simulink model "Smart_Inverter_Toolbox"  (R2024a)
settings: Solver=ode4  StartTime=0.0  StopTime=10.0  FixedStep=50e-6  RelTol=1e-3
undefined symbols (not defined in the file): DiscIntNeverNeededParam
libraries: simulink x4, spsFirstOrderFilterLib x4, spsThreePhaseSeriesRLCBranchLib x4, spsControlledVoltageSourceLib x3, spsGroundLib x2, slpidlib x2, spsabctodq0Lib x2, spsThreePhaseVIMeasurementLib x2, eeGeneralControl x1, spsdq0toabcLib x1, spsThreePhaseSourceLib x1, sps_lib x1
settings Model: Creator=Gokul_SENTRY  LastModifiedBy=Gokul_SENTRY

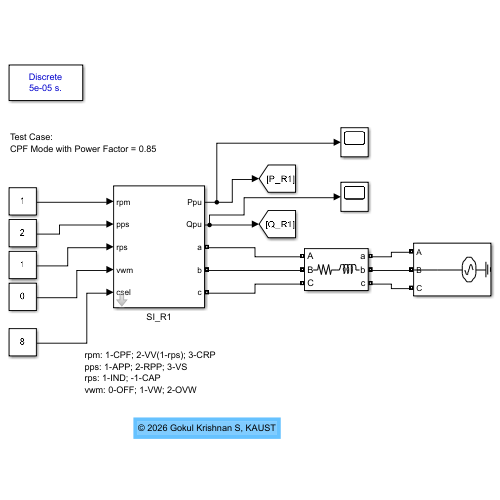
[thumbnail: Simulink's stored preview of the top-level diagram]
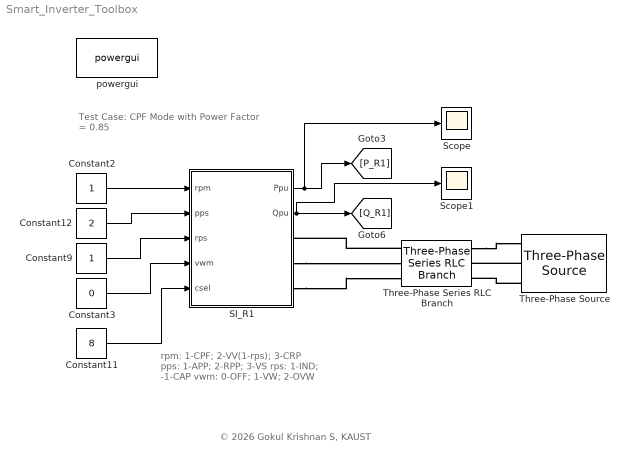
== system Smart_Inverter_Toolbox ==
  note: © 2026 Gokul Krishnan S, KAUST
  note: Test Case:
      | CPF Mode with Power Factor = 0.85
  note: rpm: 1-CPF; 2-VV(1-rps); 3-CRP
      | pps: 1-APP; 2-RPP; 3-VS
      | rps: 1-IND; -1-CAP
      | vwm: 0-OFF; 1-VW; 2-OVW
  Constant11 : Constant  Value=8
  Constant12 : Constant  Value=2
  Constant2 : Constant
  Constant3 : Constant  Value=0
  Constant9 : Constant
  SI_R1 : Subsystem  mask{Sb=10e3, Vb=400, Freq=50, rpm=CPF, pps=Active Power Priority, rps=Inductive, vwm=Off}
      mask prompts: Sb "Rated Power (VA)"; Vb "Ph-Ph RMS Voltage (V)"; Freq "Frequency (Hz)"; rpm "Reactive Power Mode"; pps "Power Priority"; rps "Reactive Power"; vwm "Volt-Watt Mode"
      mask init:
      | Idr_p = 10;      % Inductor Current Ripple in %
      | Ma    = 0.84;    % Modulation Index
      | Fsw   = 10e3;    % Inverter switching frequency (Hz)
      | Ka_p  = 20;      % Attenuation factor in %
      | 
      | Zb = (Vb^2)/Sb;
      | Cb = 1/(2*pi*Freq*Zb);
      | Vdc = (2*Vb*sqrt(2))/(Ma*sqrt(3));
      | Ib = Sb/(sqrt(3)*Vb);
      | Ib_max = Ib*sqrt(2);
      | Ir_max = Ib_max*(Idr_p/100);
      | Ka = Ka_p/100;
      | 
      | Cf = Cb*0.01;
      | 
      | L1 = Vdc/(6*Fsw*Ir_max);
      | L2 = ((sqrt(1/Ka^2))+1)/(Cf*((2*pi*Fsw)^2));
      | 
      | Fres = (1/(2*pi))*sqrt((L1+L2)/(L1*L2*Cf));
      | Rf   = 1/(3*Cf*Fres*2*pi);
      | 
      | CDC_bus = ((4*Sb)/(Vdc^2))*(1/(4*Freq));
      | 
      | PLL_Kp = -2/(Vb*sqrt(2)*(1/4)*(1/Freq));
      | PLL_Ki = PLL_Kp/(2*(1/4)*(1/Freq));
      | 
      | CC_Kp = (2*(L1+L2))/(1e-3);
      | CC_Ki = CC_Kp/(2*1e-3);
      mask TypeOptions rpm: CPF | VV | CRP
      mask TypeOptions pps: Active Power Priority | Reactive Power Priority | Vector Scaling
      mask DialogControl DescGroupVar Prompt: Smart Inverter Toolbox
      mask DialogControl DescTextVar Prompt: by Gokul, ANGLE Lab, KAUST
  Scope : Scope
  Scope1 : Scope
  Three-Phase Series RLC Branch : spsThreePhaseSeriesRLCBranchLib/Three-Phase Series RLC Branch  LConnTagsString=A|B|C  RConnTagsString=A|B|C  BranchType=RL  Resistance=1e-3  Inductance=1e-6  Capacitance=1e-6  Measurements=None
  Three-Phase Source : spsThreePhaseSourceLib/Three-Phase Source  InternalConnection=Yg  VoltagePhases=off  Voltage=400  PhaseAngle=0  Voltage_phases=[25e3 25e3 25e3]/sqrt(3)  PhaseAngles_phases=[0 -120 +120]  Frequency=50  NonIdealSource=off  SpecifyImpedance=off  Resistance=0.8929  Inductance=16.58e-3  ShortCircuitLevel=100e6  BaseVoltage=25e3  XRratio=7  BusType=swing  Pref=10e3  Qref=0  Prefabc=[10e3, 10e3, 10e3]  Qrefabc=[0, 0, 0]  Qmin=-inf  Qmax=inf
  powergui : sps_lib/powergui  Priority=1  SimulationMode=Discrete  SampleTime=50e-6  frequency=60  Iterations=50  frequencyindice=50  Pbase=100e6  ErrMax=1e-4  UnitsV=kV  UnitsW=MW  buscounter=0  FunctionMessages=off  echomessages=off  EnableUseOfTLC=off  CurrentSourceSwitches=off  DisableSnubberDevices=off  DisableRonSwitches=off  DisableVfSwitches=off  DisplayEquations=off  AutomaticDiscreteSolvers=off  SolverType=Tustin/Backward Euler (TBE)  Interpol=off  ExternalGateDelay=off  methode=off  Ts=100  x0status=blocks  SPID=on  SwTol=0  HookPort=off  NonlinearTolerance=1e-4  nMaxIteration=100  ContinueOnMaxIteration=off  RestoreLinks=warning  ResistiveCurrentMeasurement=off  Frange=[0:2:500]  Ylog=off  Xlog=on  ShowGrid=off  save=off  variable=ZData  structure=0  ZoomFFT=off  StartTime=0.0  cycles=1  DisplayStyle=1  fundamental=60  FreqAxis=off  MaxFrequency=1000  frequencyindicesteady=1  RmsSteady=1  display=off
  wires:
  Constant9/1 -> SI_R1/3(rps)
  Constant12/1 -> SI_R1/2(pps)
  SI_R1/1(Ppu) -> Scope/1, [P_R1]
  Constant3/1 -> SI_R1/4(vwm)
  Constant11/1 -> SI_R1/5(csel)
  Constant2/1 -> SI_R1/1(rpm)
  SI_R1/2(Qpu) -> Scope1/1, [Q_R1]
  connections:
  SI_R1/RConn2 -- Three-Phase Series RLC Branch/LConn2
  Three-Phase Series RLC Branch/LConn1 -- SI_R1/RConn1
  SI_R1/RConn3 -- Three-Phase Series RLC Branch/LConn3
  Three-Phase Source/RConn2 -- Three-Phase Series RLC Branch/RConn2
  Three-Phase Series RLC Branch/RConn1 -- Three-Phase Source/RConn1
  Three-Phase Source/RConn3 -- Three-Phase Series RLC Branch/RConn3

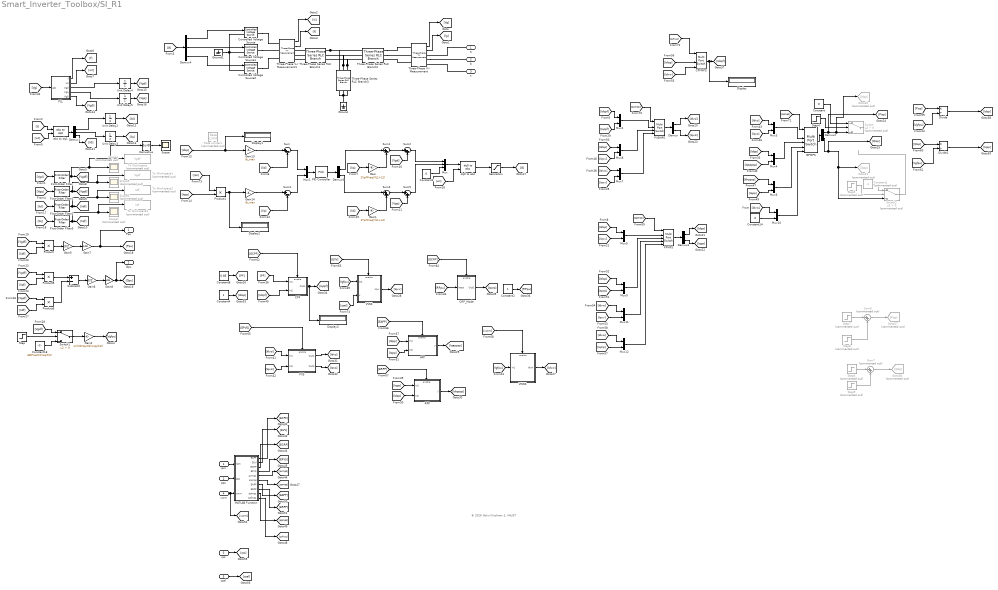
== system Smart_Inverter_Toolbox/SI_R1 ==
  note: © 2026 Gokul Krishnan S, KAUST
  rpm : Inport
  pps : Inport  Port=2
  rps : Inport  Port=3
  vwm : Inport  Port=4
  csel : Inport  Port=5
  APP : Subsystem
  CPF : Subsystem
  CPFMPS : MultiPortSwitch  DataPortOrder=Zero-based contiguous  zeroidx=on  SaturateOnIntegerOverflow=off  InputSameDT=off
  CRP_Mode : Subsystem
  Constant : Constant  Value=0
  Constant1 : Constant  Commented=on  Value=-1
  Constant14 : Constant  Value=0
  Constant18 : Constant  Value=400*sqrt(2)/sqrt(3)
  Constant2 : Constant
  Constant3 : Constant  Value=0
  Constant4 : Constant
  Constant8 : Constant  Value=0.85
  Controlled Voltage Source : spsControlledVoltageSourceLib/Controlled Voltage Source  Initialize=off  Source_Type=AC  Amplitude=0  Phase=0  Frequency=0  Measurements=None
  Controlled Voltage Source1 : spsControlledVoltageSourceLib/Controlled Voltage Source  Initialize=off  Source_Type=AC  Amplitude=0  Phase=0  Frequency=0  Measurements=None
  Controlled Voltage Source2 : spsControlledVoltageSourceLib/Controlled Voltage Source  Initialize=off  Source_Type=AC  Amplitude=0  Phase=0  Frequency=0  Measurements=None
  Demux{,2..3,9} (4 alike) : Demux  Outputs=2
  Demux1 : Demux  Outputs=3
  Demux4 : Demux  Outputs=3
  Derivative : Derivative
  Display{,1..3} (4 alike) : Display
  Divide : Product  Inputs=*/
  Divide1 : Product  Inputs=*/
  First-Order Filter : spsFirstOrderFilterLib/First-Order Filter  FilterType=Lowpass  Tc=10e-3  Ts=0  Initialize=on  Vac_Init=[((Vb*sqrt(2))/sqrt(3)), 0, Freq]  Vdc_Init=0  PlotResponse=off  FreqRange="[0,  200,  1]"
  First-Order Filter1 : spsFirstOrderFilterLib/First-Order Filter  FilterType=Lowpass  Tc=10e-3  Ts=0  Initialize=on  Vac_Init=[0, 0, Freq]  Vdc_Init=0  PlotResponse=off  FreqRange="[0,  200,  1]"
  First-Order Filter2 : spsFirstOrderFilterLib/First-Order Filter  FilterType=Lowpass  Tc=10e-3  Ts=0  Initialize=on  Vac_Init=[0, 0, Freq]  Vdc_Init=0  PlotResponse=off  FreqRange="[0,  200,  1]"
  First-Order Filter3 : spsFirstOrderFilterLib/First-Order Filter  FilterType=Lowpass  Tc=10e-3  Ts=0  Initialize=on  Vac_Init=[0, 0, Freq]  Vdc_Init=0  PlotResponse=off  FreqRange="[0,  200,  1]"
  Gain : Gain  Gain=2*pi*Freq*(L1+L2)
  Gain1 : Gain  Gain=2*pi*Freq*(L1+L2)
  Gain13 : Gain  Gain=Ib_max
  Gain14 : Gain  Gain=Ib_max
  Gain2 : Gain  Gain=1/((Vb*sqrt(2))/sqrt(3))
  Gain5 : Gain  Gain=3/2
  Gain6 : Gain  Gain=3/2
  Gain7 : Gain  Gain=1/Sb
  Gain8 : Gain  Gain=1/Sb
  Goto40 : Goto  Commented=on  GotoTag=Idsp
  Goto41 : Goto  Commented=on  GotoTag=Iqsp
  Goto57 : Goto  Commented=on  GotoTag=Pisp
  Goto58 : Goto  Commented=on  GotoTag=Qisp
  Ground : spsGroundLib/Ground  LConnTagsString=a
  Ground1 : spsGroundLib/Ground  LConnTagsString=a
  ISPMPS : MultiPortSwitch  DataPortOrder=Zero-based contiguous  Inputs=5  zeroidx=on  SaturateOnIntegerOverflow=off  InputSameDT=off
  MATLAB Function : MATLAB Function  TreatAsAtomicUnit=on
  Mux : Mux  Inputs=3
  Mux{1..12} (12 alike) : Mux  Inputs=2
  PID Controller : slpidlib/PID Controller  Controller=PI  Form=Parallel  TimeDomain=Continuous-time  UseExternalTs=off  SampleTime=-1  IntegratorMethod=Forward Euler  FilterMethod=Forward Euler  ControllerParametersSource=internal  P=CC_Kp  I=CC_Ki  UseKiTs=off  D=0  UseExternalDerivativeSource=off  N=100  UseFilter=on  TunerSelectOption=Transfer Function Based (PID Tuner App)  InitialConditionSource=internal  InitialConditionForIntegrator=0  InitialConditionForFilter=0  DifferentiatorICPrevScaledInput=0  ExternalReset=none  TrackingMode=off  Kt=1  LimitOutput=off  SatLimitsSource=internal  UpperSaturationLimit=inf  LowerSaturationLimit=-inf  LinearizeAsGain=on  AntiWindupMode=none  Kb=1  LimitIntegrator=off  UpperIntegratorSaturationLimit=inf  LowerIntegratorSaturationLimit=-inf  POutMin=[]  POutMax=[]  IOutMin=[]  IOutMax=[]  DOutMin=[]  DOutMax=[]  NOutMin=[]  NOutMax=[]  SumOutMin=[]  SumOutMax=[]  SaturationOutMin=[]  SaturationOutMax=[]  PParamMin=[]  PParamMax=[]  IParamMin=[]  IParamMax=[]  DParamMin=[]  DParamMax=[]  NParamMin=[]  NParamMax=[]  KbParamMin=[]  KbParamMax=[]  KtParamMin=[]  KtParamMax=[]  KbOutMin=[]  KbOutMax=[]  KtOutMin=[]  KtOutMax=[]  IntegratorOutMin=[]  IntegratorOutMax=[]  FilterOutMin=[]  FilterOutMax=[]  SumI1OutMin=[]  SumI1OutMax=[]  SumI2OutMin=[]  SumI2OutMax=[]  SumI3OutMin=[]  SumI3OutMax=[]  SumI4OutMin=[]  SumI4OutMax=[]  SumDOutMin=[]  SumDOutMax=[]  DifferentiatorOutMin=[]  DifferentiatorOutMax=[]  FilterDiffOutCoefMin=[]  FilterDiffOutCoefMax=[]  ReciprocalOutMin=[]  ReciprocalOutMax=[]  SumDenOutMin=[]  SumDenOutMax=[]  SumNumOutMin=[]  SumNumOutMax=[]  DivideOutMin=[]  DivideOutMax=[]  UdiffTsProdOutMin=[]  UdiffTsProdOutMax=[]  NTsProdOutMin=[]  NTsProdOutMax=[]  UintegralTsProdOutMin=[]  UintegralTsProdOutMax=[]  UngainTsProdOutMin=[]  UngainTsProdOutMax=[]  ClampingZeroOutDataTypeStr=Inherit: Inherit via back propagation  ClampingZeroOutMin=[]  ClampingZeroOutMax=[]  FilterDenConstantOutDataTypeStr=Inherit: Inherit via back propagation  FilterDenConstantOutMin=[]  FilterDenConstantOutMax=[]  PCopyOutDataTypeStr=Inherit: Inherit via back propagation  PCopyOutMin=[]  PCopyOutMax=[]  NCopyOutDataTypeStr=Inherit: Inherit via back propagation  NCopyOutMin=[]  NCopyOutMax=[]  IntegratorContinuousStateAttributes=''  IntegratorStateMustResolveToSignalObject=off  IntegratorRTWStateStorageClass=Auto  FilterContinuousStateAttributes=''  FilterStateMustResolveToSignalObject=off  FilterRTWStateStorageClass=Auto  ParallelPVariant=InternalParameters  IdealPVariant=Disabled  IVariant=InternalParameters  DVariant=Disabled  IntegratorVariant=Continuous  SatVariant=Disabled  AWVariant=Passthrough  PCopyVariant=Disabled  TRVariant=Disabled  FdbkBlocksVariant=Forward  IdealPFdbkVariant=Disabled  SatFdbkVariant=Disabled  DerivativeFilterVariant=Disabled  NVariant=Disabled  NCopyVariant=Disabled_SignalSpec  FilterICVariant=Disabled  IntegratorICVariant=InternalICs  ExternalResetVariant=Disabled  TRSumVariant=Passthrough  SumFdbkVariant=Disabled  SumVariant=Sum_PI  TsampFilterVariant=InternalTs  TsampNgainVariant=Passthrough  TsampIntegralVariant=Disabled_SignalSpec  ExternalSaturationOutDataTypeStr=Inherit: Same as second input  DerivativeSourceVariant=Disabled
  PLL : Subsystem
  PPMPS : MultiPortSwitch  DataPortOrder=Zero-based contiguous  Inputs=5  zeroidx=on  SaturateOnIntegerOverflow=off  InputSameDT=off
  PVS : Subsystem
  PVSMPS : MultiPortSwitch  DataPortOrder=Zero-based contiguous  Inputs=4  zeroidx=on  SaturateOnIntegerOverflow=off  InputSameDT=off
  Product{,1,5..6} (4 alike) : Product
  RPP : Subsystem
  Rate Limiter1 : RateLimiter  Commented=on  RisingSlewLimit=2  FallingSlewLimit=-2  SampleTimeMode=inherited
  Saturation : Saturate  UpperLimit=Vb*1.2*sqrt(2)/sqrt(3)  LowerLimit=-1*1.2*Vb*sqrt(2)/sqrt(3)
  Scope : Scope
  Scope{4..7} (4 alike) : Scope  Commented=on
  Step : Step  Time=0.1  SampleTime=0
  Step4 : Step  Time=7.05  SampleTime=0
  Step5 : Step  Commented=on  Time=7.05  SampleTime=0
  Step6 : Step  Commented=on  Time=3  Before=0.2  After=0.1  SampleTime=0
  Step7 : Step  Commented=on  Time=2  Before=0.9  After=0.8  SampleTime=0
  Step8 : Step  Commented=on  Time=2.5  After=+0.1  SampleTime=0
  Step9 : Step  Commented=on  Time=3.5  After=0.1  SampleTime=0
  Subtract2 : Sum  Inputs=+-
  Sum : Sum  Inputs=|+-
  Sum1 : Sum  Inputs=|+-
  Sum2 : Sum  Inputs=|++
  Sum3 : Sum  Inputs=|+-
  Sum4 : Sum  Inputs=|++
  Sum5 : Sum  Inputs=|++
  Sum6 : Sum  Commented=on  Inputs=|++
  Sum7 : Sum  Commented=on  Inputs=|++
  Switch : Switch  Commented=on  Criteria=u2 > Threshold  SaturateOnIntegerOverflow=off  InputSameDT=off
  Switch1 : Switch  Criteria=u2 > Threshold  SaturateOnIntegerOverflow=off  InputSameDT=off
  Switch2 : Switch  Commented=on  Criteria=u2 > Threshold  SaturateOnIntegerOverflow=off  InputSameDT=off
  Three-Phase Series RLC Branch1 : spsThreePhaseSeriesRLCBranchLib/Three-Phase Series RLC Branch  LConnTagsString=A|B|C  RConnTagsString=A|B|C  BranchType=L  Resistance=1  Inductance=L1  Capacitance=1e-6  Measurements=None
  Three-Phase Series RLC Branch2 : spsThreePhaseSeriesRLCBranchLib/Three-Phase Series RLC Branch  LConnTagsString=A|B|C  RConnTagsString=A|B|C  BranchType=L  Resistance=1  Inductance=L2  Capacitance=1e-6  Measurements=None
  Three-Phase Series RLC Branch3 : spsThreePhaseSeriesRLCBranchLib/Three-Phase Series RLC Branch  LConnTagsString=A|B|C  RConnTagsString=A|B|C  BranchType=RC  Resistance=Rf  Inductance=1e-3  Capacitance=Cf  Measurements=None
  Three-Phase V-I Measurement : spsThreePhaseVIMeasurementLib/Three-Phase V-I Measurement  VoltageMeasurement=phase-to-ground  SetLabelV=off  LabelV=Vabc  Vpu=off  VpuLL=off  CurrentMeasurement=yes  SetLabelI=off  LabelI=Iabc  Ipu=off  Pbase=100e6  Vbase=500e3  OutputType=Complex  PhasorSimulation=off  PSBequivalent=0
  Three-Phase V-I Measurement1 : spsThreePhaseVIMeasurementLib/Three-Phase V-I Measurement  VoltageMeasurement=phase-to-ground  SetLabelV=off  LabelV=Vabc  Vpu=off  VpuLL=off  CurrentMeasurement=yes  SetLabelI=off  LabelI=Iabc  Ipu=off  Pbase=100e6  Vbase=500e3  OutputType=Complex  PhasorSimulation=off  PSBequivalent=0
  To Workspace : ToWorkspace  Commented=on  VariableName=Vgdf  SaveFormat=Timeseries  SampleTime=-1
  To Workspace1 : ToWorkspace  Commented=on  VariableName=Vgqf  SaveFormat=Timeseries  SampleTime=-1
  To Workspace2 : ToWorkspace  Commented=on  VariableName=Iidf  SaveFormat=Timeseries  SampleTime=-1
  To Workspace3 : ToWorkspace  Commented=on  VariableName=Iiqf  SaveFormat=Timeseries  SampleTime=-1
  Unit Delay{2..5} (4 alike) : UnitDelay  SampleTime=-1  HasFrameUpgradeWarning=on
  VVSS : Subsystem
  VWSS : Subsystem
  abc to dq1 : spsabctodq0Lib/abc to dq0  Alignment=90 degrees behind phase A axis
  dq0 to abc : spsdq0toabcLib/dq0 to abc  Alignment=90 degrees behind phase A axis
  a : PMIOPort  Side=Right
  b : PMIOPort  Port=2  Side=Right
  c : PMIOPort  Port=3  Side=Right
  Ppu : Outport
  Qpu : Outport  Port=2
  wires:
  PLL/2(wt) -> [wt]
  [Iqsp] -> Product1/2
  Product1/1 -> Display2/1, Gain14/1
  MATLAB Function/10(cpfmps) -> [cpfmps]
  MATLAB Function/9(ppmps) -> [ppmps]
  MATLAB Function/8(ERPP) -> [ERPP]
  MATLAB Function/7(EAPP) -> [EAPP]
  MATLAB Function/6(spmps) -> [spmps]
  MATLAB Function/5(pvmps) -> [pvmps]
  MATLAB Function/4(EPVS) -> [EPVS]
  MATLAB Function/3(ECRP) -> [ECRP]
  MATLAB Function/2(EVV) -> [EVV]
  MATLAB Function/1(ECPF) -> [ECPF]
  vwm/1 -> MATLAB Function/3(vwm), [vwm]
  pps/1 -> MATLAB Function/2(pps)
  rpm/1 -> MATLAB Function/1(rpm)
  [Idsp] -> Display1/1, Gain13/1
  [Vgfpu] -> Divide/2
  Constant18/1 -> Switch1/3
  Step/1 -> Switch1/2
  [Vgdf] -> Switch1/1
  Switch1/1 -> Gain2/1
  [Vgfpu] -> Divide1/2
  [Qisp] -> Divide1/1
  [Pisp] -> Divide/1
  Saturation/1 -> [G]
  dq0 to abc/1 -> Saturation/1
  [Iqcrp] -> Mux12/2
  [Idvw] -> Mux12/1
  Mux12/1 -> PPMPS/6
  Unit Delay5/1 -> [Vgq]
  Unit Delay4/1 -> [Vgd]
  Unit Delay3/1 -> [Iiq]
  Unit Delay2/1 -> [Iid]
  [EPVS] -> PVS/Enable
  [ERPP] -> RPP/Enable
  [EAPP] -> APP/Enable
  [Idvw] -> CPFMPS/4
  [Idisp] -> CPFMPS/3
  [cpfmps] -> CPFMPS/1
  CPFMPS/1 -> Display/1, [Idcpf]
  Demux/1 -> [Idvsi]
  Mux7/1 -> PVSMPS/5
  [Iqvv] -> Mux7/2
  [Idvw] -> Mux7/1
  Mux11/1 -> PPMPS/5
  [Idvw] -> Mux11/1
  [Iqvv] -> Mux11/2
  Constant14/1 -> Mux10/2
  [Idvw] -> Mux10/1
  Mux10/1 -> ISPMPS/6
  Constant2/1 -> [RPpu]
  [Iqcrp] -> Mux9/2
  [Idisp] -> Mux9/1
  Mux9/1 -> PPMPS/4
  [vwm] -> VWSS/Enable
  [ECRP] -> CRP_Mode/Enable
  [EVV] -> VVSS/Enable
  [ECPF] -> CPF/Enable
  Mux5/1 -> PPMPS/3
  Mux6/1 -> ISPMPS/5
  Mux4/1 -> ISPMPS/4
  Mux3/1 -> ISPMPS/3
  Mux2/1 -> PVSMPS/3
  Mux8/1 -> PVSMPS/4
  [Idisp] -> Mux8/1
  [Iqvv] -> Mux8/2
  [Idrppsp] -> Mux6/1
  [Iqpp] -> Mux6/2
  [Iqvv] -> Mux5/2
  [Idisp] -> Mux5/1
  Demux3/2 -> [Iqpp]
  Demux3/1 -> [Idpp]
  PPMPS/1 -> Demux3/1
  [ppmps] -> PPMPS/1
  [Iqappsp] -> Mux4/2
  [Idpp] -> Mux4/1
  Constant4/1 -> [Idisp]
  Constant8/1 -> [PF]
  [spmps] -> ISPMPS/1
  ISPMPS/1 -> Demux2/1
  [Idvs] -> Mux3/1
  [Iqvs] -> Mux3/2
  [Iqcpf] -> Mux2/2
  [Idcpf] -> Mux2/1
  Demux/2 -> [Iqvsi]
  PVSMPS/1 -> Demux/1
  [pvmps] -> PVSMPS/1
  Gain5/1 -> Gain7/1
  [Iqpp] -> APP/2(In2)
  [Iqvsi] -> PVS/2(In2)
  [RPpu] -> CRP_Mode/1(Input)
  Gain8/1 -> [Qpu], Qpu/1
  First-Order Filter1/1 -> To Workspace1/1, Scope5/1, [Vgqf]
  VWSS/1(Idvw) -> [Idvw]
  Gain7/1 -> [Ppu], Ppu/1
  [wt] -> dq0 to abc/2
  [Vgdf] -> Product5/1
  PLL/4(Vgq) -> Unit Delay5/1
  PLL/5(Vg0) -> [Vg0]
  Three-Phase V-I Measurement/2 -> [Ig]
  Demux4/2 -> Controlled Voltage Source1/1
  [Vgq] -> First-Order Filter1/1
  [Idcpf] -> CPF/2(In2)
  CPF/1(Out1) -> Display3/1, [Iqcpf]
  First-Order Filter3/1 -> To Workspace3/1, Scope7/1, [Iiqf]
  [Vgfpu] -> VVSS/1(In1)
  [Idpp] -> APP/1(In1)
  [Iqpp] -> RPP/1(In1)
  APP/1(y) -> [Iqappsp]
  [Idpp] -> RPP/2(In2)
  [Iidf] -> Product6/2
  Gain6/1 -> Gain8/1
  First-Order Filter/1 -> Derivative/1, To Workspace/1, Scope4/1, [Vgdf]
  First-Order Filter2/1 -> To Workspace2/1, Scope6/1, [Iidf]
  [Iiqf] -> Product5/2
  PID Controller/1 -> Demux9/1
  Subtract2/1 -> Gain6/1
  CRP_Mode/1(Out1) -> [Iqcrp]
  [Iiq] -> Gain/1
  Product5/1 -> Subtract2/1
  [Vgfpu] -> VWSS/1(In1)
  Gain2/1 -> [Vgfpu]
  [Iiq] -> First-Order Filter3/1
  Sum/1 -> Mux1/1
  Three-Phase V-I Measurement/1 -> [Vg]
  Demux4/1 -> Controlled Voltage Source/1
  [Vgd] -> First-Order Filter/1
  [Vg] -> PLL/1(abc)
  Sum5/1 -> Mux/2
  [Vgq] -> Sum5/2
  PVS/2(Out2) -> [Iqvs]
  [Iid] -> Gain1/1
  Gain13/1 -> Sum/1
  Three-Phase V-I Measurement1/2 -> [Ii]
  RPP/1(y) -> [Idrppsp]
  [Iiq] -> Sum3/2
  Mux1/1 -> PID Controller/1
  [Ii] -> abc to dq1/1
  Demux1/2 -> Unit Delay3/1
  [Vgqf] -> Product6/1
  [Vgdf] -> Product/1
  Constant3/1 -> Mux/3
  abc to dq1/1 -> Demux1/1
  [G] -> Demux4/1
  [Iidf] -> Product/2
  Demux1/3 -> [Ii0]
  Mux/1 -> dq0 to abc/1
  Product6/1 -> Subtract2/2
  PVS/1(Out1) -> [Idvs]
  Sum1/1 -> Sum2/1
  [wt] -> abc to dq1/2
  [Idvsi] -> PVS/1(In1)
  Demux9/1 -> Sum1/1
  Sum2/1 -> Mux/1
  VVSS/1(Iqvv) -> [Iqvv]
  PLL/1(f) -> [f]
  Gain/1 -> Sum1/2
  Demux1/1 -> Unit Delay2/1
  Product/1 -> Gain5/1
  Demux9/2 -> Sum4/1
  [PF] -> CPF/1(In1)
  [Iid] -> Sum/2
  Sum4/1 -> Sum5/1
  [Iid] -> First-Order Filter2/1
  Gain1/1 -> Sum4/2
  PLL/3(Vgd) -> Unit Delay4/1
  [Vgd] -> Sum2/2
  Three-Phase V-I Measurement1/1 -> [Vi]
  Sum3/1 -> Mux1/2
  Demux4/3 -> Controlled Voltage Source2/1
  Divide/1 -> [Idsp]
  Divide1/1 -> [Iqsp]
  Derivative/1 -> Scope/1
  Gain14/1 -> Sum3/1
  Demux2/2 -> [Qisp], Switch2/3, Goto41/1
  Demux2/1 -> [Pisp], Switch/3, Goto40/1
  Constant/1 -> Switch/1
  Step4/1 -> Switch/2
  Step5/1 -> Switch2/2
  Switch2/1 -> ?
  Constant1/1 -> Switch2/1
  [rps] -> Product1/1
  rps/1 -> [rps]
  csel/1 -> [csel]
  [csel] -> VVSS/2(x)
  Sum7/1 -> Goto58/1
  Step8/1 -> Sum6/2
  Step9/1 -> Sum7/2
  Sum6/1 -> Goto57/1
  Step7/1 -> Sum6/1
  Step6/1 -> Sum7/1
  connections:
  Three-Phase V-I Measurement/RConn2 -- b/RConn1
  c/RConn1 -- Three-Phase V-I Measurement/RConn3
  Controlled Voltage Source1/LConn1 -- Controlled Voltage Source2/LConn1 -- Controlled Voltage Source/LConn1 -- Ground1/LConn1
  Three-Phase Series RLC Branch1/LConn2 -- Three-Phase V-I Measurement1/RConn2
  Three-Phase Series RLC Branch1/RConn1 -- Three-Phase Series RLC Branch3/LConn1 -- Three-Phase Series RLC Branch2/LConn1
  Three-Phase Series RLC Branch1/LConn1 -- Three-Phase V-I Measurement1/RConn1
  Three-Phase Series RLC Branch1/LConn3 -- Three-Phase V-I Measurement1/RConn3
  Three-Phase V-I Measurement/LConn3 -- Three-Phase Series RLC Branch2/RConn3
  Three-Phase Series RLC Branch2/RConn1 -- Three-Phase V-I Measurement/LConn1
  Controlled Voltage Source1/RConn1 -- Three-Phase V-I Measurement1/LConn2
  Three-Phase Series RLC Branch2/RConn2 -- Three-Phase V-I Measurement/LConn2
  Controlled Voltage Source2/RConn1 -- Three-Phase V-I Measurement1/LConn3
  a/RConn1 -- Three-Phase V-I Measurement/RConn1
  Three-Phase Series RLC Branch3/LConn2 -- Three-Phase Series RLC Branch1/RConn2 -- Three-Phase Series RLC Branch2/LConn2
  Controlled Voltage Source/RConn1 -- Three-Phase V-I Measurement1/LConn1
  Three-Phase Series RLC Branch3/LConn3 -- Three-Phase Series RLC Branch1/RConn3 -- Three-Phase Series RLC Branch2/LConn3
  Three-Phase Series RLC Branch3/RConn2 -- Ground/LConn1 -- Three-Phase Series RLC Branch3/RConn3 -- Three-Phase Series RLC Branch3/RConn1

== system Smart_Inverter_Toolbox/SI_R1/APP ==
  In1 : Inport
  In2 : Inport  Port=2
  Enable : EnablePort
  APP : simulink/Discontinuities/Saturation Dynamic  OutMin=[]  OutMax=[]  OutDataTypeStr=Inherit: Same as second input  OutDataType=fixdt(1, 16)  OutScaling=2^-10  DoSatur=off
  Constant25 : Constant
  Constant26 : Constant  Value=0
  Gain10 : Gain  Gain=-1
  Max2 : MinMax  Function=max  Inputs=2
  Square : Math  Operator=square
  Square Root : Sqrt
  Square1 : Math  Operator=square
  Subtract : Sum  Inputs=+-
  y : Outport
  wires:
  In1/1 -> Square1/1
  Subtract/1 -> Max2/1
  Square Root/1 -> Gain10/1, APP/1
  Constant26/1 -> Max2/2
  Max2/1 -> Square Root/1
  Square1/1 -> Subtract/2
  Gain10/1 -> APP/3
  In2/1 -> APP/2
  Square/1 -> Subtract/1
  APP/1 -> y/1
  Constant25/1 -> Square/1

== system Smart_Inverter_Toolbox/SI_R1/CPF ==
  In1 : Inport
  In2 : Inport  Port=2
  Enable : EnablePort
  Acos : Trigonometry  Operator=acos
  Product3 : Product
  Tan : Trigonometry  Operator=tan
  Out1 : Outport
  wires:
  Product3/1 -> Out1/1
  In1/1 -> Acos/1
  Tan/1 -> Product3/1
  In2/1 -> Product3/2
  Acos/1 -> Tan/1

== system Smart_Inverter_Toolbox/SI_R1/CRP_Mode ==
  Input : Inport
  Enable : EnablePort
  Constant2 : Constant
  Max1 : MinMax  Inputs=2
  Out1 : Outport
  wires:
  Max1/1 -> Out1/1
  Input/1 -> Max1/1
  Constant2/1 -> Max1/2

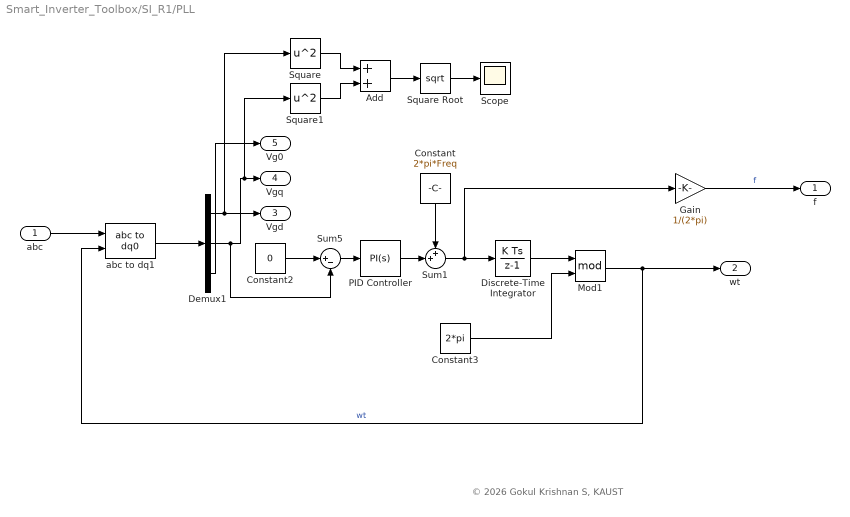
== system Smart_Inverter_Toolbox/SI_R1/PLL ==
  note: © 2026 Gokul Krishnan S, KAUST
  abc : Inport
  Add : Sum
  Constant : Constant  Value=2*pi*Freq
  Constant2 : Constant  Value=0
  Constant3 : Constant  Value=2*pi
  Demux1 : Demux  Outputs=3
  Discrete-Time Integrator : DiscreteIntegrator  SampleTime=-1  ICPrevOutput=DiscIntNeverNeededParam  ICPrevScaledInput=DiscIntNeverNeededParam
  Gain : Gain  Gain=1/(2*pi)
  Mod1 : Math  Operator=mod
  PID Controller : slpidlib/PID Controller  Controller=PI  Form=Parallel  TimeDomain=Continuous-time  UseExternalTs=off  SampleTime=-1  IntegratorMethod=Forward Euler  FilterMethod=Forward Euler  ControllerParametersSource=internal  P=PLL_Kp  I=PLL_Ki  UseKiTs=off  D=0  UseExternalDerivativeSource=off  N=100  UseFilter=on  TunerSelectOption=Transfer Function Based (PID Tuner App)  InitialConditionSource=internal  InitialConditionForIntegrator=0  InitialConditionForFilter=0  DifferentiatorICPrevScaledInput=0  ExternalReset=none  TrackingMode=off  Kt=1  LimitOutput=off  SatLimitsSource=internal  UpperSaturationLimit=inf  LowerSaturationLimit=-inf  LinearizeAsGain=on  AntiWindupMode=none  Kb=1  LimitIntegrator=off  UpperIntegratorSaturationLimit=inf  LowerIntegratorSaturationLimit=-inf  POutMin=[]  POutMax=[]  IOutMin=[]  IOutMax=[]  DOutMin=[]  DOutMax=[]  NOutMin=[]  NOutMax=[]  SumOutMin=[]  SumOutMax=[]  SaturationOutMin=[]  SaturationOutMax=[]  PParamMin=[]  PParamMax=[]  IParamMin=[]  IParamMax=[]  DParamMin=[]  DParamMax=[]  NParamMin=[]  NParamMax=[]  KbParamMin=[]  KbParamMax=[]  KtParamMin=[]  KtParamMax=[]  KbOutMin=[]  KbOutMax=[]  KtOutMin=[]  KtOutMax=[]  IntegratorOutMin=[]  IntegratorOutMax=[]  FilterOutMin=[]  FilterOutMax=[]  SumI1OutMin=[]  SumI1OutMax=[]  SumI2OutMin=[]  SumI2OutMax=[]  SumI3OutMin=[]  SumI3OutMax=[]  SumI4OutMin=[]  SumI4OutMax=[]  SumDOutMin=[]  SumDOutMax=[]  DifferentiatorOutMin=[]  DifferentiatorOutMax=[]  FilterDiffOutCoefMin=[]  FilterDiffOutCoefMax=[]  ReciprocalOutMin=[]  ReciprocalOutMax=[]  SumDenOutMin=[]  SumDenOutMax=[]  SumNumOutMin=[]  SumNumOutMax=[]  DivideOutMin=[]  DivideOutMax=[]  UdiffTsProdOutMin=[]  UdiffTsProdOutMax=[]  NTsProdOutMin=[]  NTsProdOutMax=[]  UintegralTsProdOutMin=[]  UintegralTsProdOutMax=[]  UngainTsProdOutMin=[]  UngainTsProdOutMax=[]  ClampingZeroOutDataTypeStr=Inherit: Inherit via back propagation  ClampingZeroOutMin=[]  ClampingZeroOutMax=[]  FilterDenConstantOutDataTypeStr=Inherit: Inherit via back propagation  FilterDenConstantOutMin=[]  FilterDenConstantOutMax=[]  PCopyOutDataTypeStr=Inherit: Inherit via back propagation  PCopyOutMin=[]  PCopyOutMax=[]  NCopyOutDataTypeStr=Inherit: Inherit via back propagation  NCopyOutMin=[]  NCopyOutMax=[]  IntegratorContinuousStateAttributes=''  IntegratorStateMustResolveToSignalObject=off  IntegratorRTWStateStorageClass=Auto  FilterContinuousStateAttributes=''  FilterStateMustResolveToSignalObject=off  FilterRTWStateStorageClass=Auto  ParallelPVariant=InternalParameters  IdealPVariant=Disabled  IVariant=InternalParameters  DVariant=Disabled  IntegratorVariant=Continuous  SatVariant=Disabled  AWVariant=Passthrough  PCopyVariant=Disabled  TRVariant=Disabled  FdbkBlocksVariant=Forward  IdealPFdbkVariant=Disabled  SatFdbkVariant=Disabled  DerivativeFilterVariant=Disabled  NVariant=Disabled  NCopyVariant=Disabled_SignalSpec  FilterICVariant=Disabled  IntegratorICVariant=InternalICs  ExternalResetVariant=Disabled  TRSumVariant=Passthrough  SumFdbkVariant=Disabled  SumVariant=Sum_PI  TsampFilterVariant=InternalTs  TsampNgainVariant=Passthrough  TsampIntegralVariant=Disabled_SignalSpec  ExternalSaturationOutDataTypeStr=Inherit: Same as second input  DerivativeSourceVariant=Disabled
  Scope : Scope
  Square : Math  Operator=square
  Square Root : Sqrt
  Square1 : Math  Operator=square
  Sum1 : Sum  Inputs=++|
  Sum5 : Sum  Inputs=|+-
  abc to dq1 : spsabctodq0Lib/abc to dq0  Alignment=90 degrees behind phase A axis
  f : Outport
  wt : Outport  Port=2
  Vgd : Outport  Port=3
  Vgq : Outport  Port=4
  Vg0 : Outport  Port=5
  wires:
  Square Root/1 -> Scope/1
  Add/1 -> Square Root/1
  Square1/1 -> Add/2
  Square/1 -> Add/1
  Constant2/1 -> Sum5/1
  Demux1/1 -> Vgd/1, Square/1
  Constant/1 -> Sum1/1
  Sum1/1 -> Discrete-Time Integrator/1, Gain/1
  PID Controller/1 -> Sum1/2
  Discrete-Time Integrator/1 -> Mod1/1
  Mod1/1 -> wt/1, abc to dq1/2  "wt"
  Demux1/2 -> Vgq/1, Square1/1, Sum5/2
  abc to dq1/1 -> Demux1/1
  Sum5/1 -> PID Controller/1
  Constant3/1 -> Mod1/2
  Demux1/3 -> Vg0/1
  abc/1 -> abc to dq1/1
  Gain/1 -> f/1  "f"

== system Smart_Inverter_Toolbox/SI_R1/PVS ==
  In1 : Inport
  In2 : Inport  Port=2
  Enable : EnablePort
  Add : Sum
  Constant29 : Constant
  Divide2 : Product  Inputs=*/
  Min : MinMax  Inputs=2
  Product1 : Product
  Product2 : Product
  Square Root2 : Sqrt
  Square4 : Math  Operator=square
  Square5 : Math  Operator=square
  Out1 : Outport
  Out2 : Outport  Port=2
  wires:
  Product2/1 -> Out2/1
  Product1/1 -> Out1/1
  Min/1 -> Product1/2, Product2/1
  Square5/1 -> Add/2
  In2/1 -> Square5/1, Product2/2
  Square4/1 -> Add/1
  Add/1 -> Square Root2/1
  Constant29/1 -> Divide2/1, Min/1
  Divide2/1 -> Min/2
  Square Root2/1 -> Divide2/2
  In1/1 -> Square4/1, Product1/1

== system Smart_Inverter_Toolbox/SI_R1/RPP ==
  In1 : Inport
  In2 : Inport  Port=2
  Enable : EnablePort
  Constant27 : Constant
  Constant28 : Constant  Value=0
  Gain11 : Gain  Gain=-1
  Max3 : MinMax  Function=max  Inputs=2
  RPP : simulink/Discontinuities/Saturation Dynamic  OutMin=[]  OutMax=[]  OutDataTypeStr=Inherit: Same as second input  OutDataType=fixdt(1, 16)  OutScaling=2^-10  DoSatur=off
  Square Root1 : Sqrt
  Square2 : Math  Operator=square
  Square3 : Math  Operator=square
  Subtract1 : Sum  Inputs=+-
  y : Outport
  wires:
  RPP/1 -> y/1
  In1/1 -> Square3/1
  Constant27/1 -> Square2/1
  Square2/1 -> Subtract1/1
  Square Root1/1 -> RPP/1, Gain11/1
  In2/1 -> RPP/2
  Max3/1 -> Square Root1/1
  Square3/1 -> Subtract1/2
  Subtract1/1 -> Max3/1
  Constant28/1 -> Max3/2
  Gain11/1 -> RPP/3

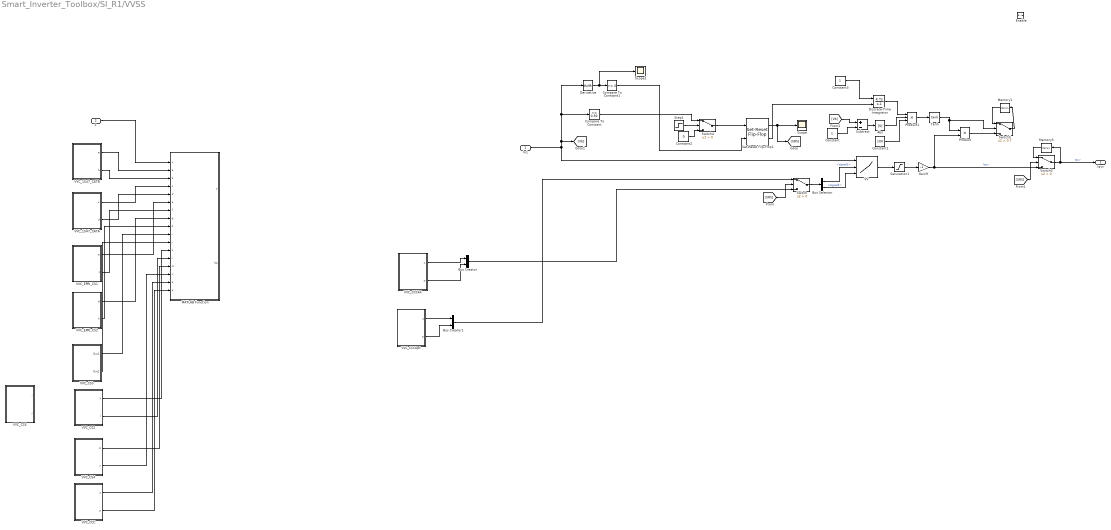
== system Smart_Inverter_Toolbox/SI_R1/VVSS ==
  In1 : Inport
  x : Inport  Port=2
  Enable : EnablePort
  Abs : Abs  SaturateOnIntegerOverflow=off
  Bus Creator : BusCreator  Inputs=2
  Bus Creator1 : BusCreator  Inputs=2
  Bus Selector : BusSelector  OutputSignals=signal1,signal2
  Compare To Constant : simulink/Logic and Bit Operations/Compare To Constant  relop=<=  const=0.92  OutDataTypeStr=boolean
  Compare To Constant1 : simulink/Logic and Bit Operations/Compare To Constant  relop=>=  const=4  OutDataTypeStr=boolean
  Constant : Constant
  Constant1 : Constant  Value=100
  Constant2 : Constant  Value=0
  Constant3 : Constant
  Derivative : Derivative
  Discrete-Time Integrator : DiscreteIntegrator  ExternalReset=level  SampleTime=-1  ICPrevOutput=DiscIntNeverNeededParam  ICPrevScaledInput=DiscIntNeverNeededParam
  Gain9 : Gain  Gain=-1
  MATLAB Function : MATLAB Function  TreatAsAtomicUnit=on
  Memory1 : Memory
  Memory3 : Memory
  Product : Product
  Product1 : Product  Inputs=3
  Saturation1 : Saturate  UpperLimit=1  LowerLimit=-1
  Scope : Scope
  Scope1 : Scope
  Set-Reset Flip-Flop1 : eeGeneralControl/Set-Reset Flip-Flop  LabelModeActiveChoice=Discrete  UndefState=Set  Q0=0  Ts=-1
      settings: LibrarySourceBlock=ee_sl_lib/General Control/Set-Reset Flip-Flop
  Step1 : Step  Time=2  SampleTime=0
  Subtract : Sum  Inputs=+-
  Switch : Switch  Criteria=u2 > Threshold  SaturateOnIntegerOverflow=off  InputSameDT=off
  Switch3 : Switch  Criteria=u2 > Threshold  SaturateOnIntegerOverflow=off  InputSameDT=off
  Switch4 : Switch  Criteria=u2 > Threshold  SaturateOnIntegerOverflow=off  InputSameDT=off
  Switch5 : Switch  Criteria=u2 > Threshold  Threshold=0.7  SaturateOnIntegerOverflow=off  InputSameDT=off
  Tanh : Trigonometry  Operator=tanh
  VV : Lookup_n-D  NumberOfTableDimensions=1  BreakpointsForDimension1Source=Input port  BreakpointsForDimension1=[-5:5]  TableSource=Input port  Table=tanh([-5:5])  ExtrapMethod=Clip  InternalRulePriority=Speed  RndMeth=Simplest
      settings: InputPortMap=u0,p221,p5
  VVC_1547_CATA : Subsystem
  VVC_1547_CATB : Subsystem
  VVC_CCC : Subsystem
  VVC_CCC44 : Subsystem
  VVC_CCCOpt : Subsystem
  VVC_CS2 : Subsystem
  VVC_CS3 : Subsystem
  VVC_CS4 : Subsystem
  VVC_CS5 : Subsystem
  VVC_EPRI_CS1 : Subsystem
  VVC_EPRI_CS2 : Subsystem
  Iqvv : Outport
  wires:
  x/1 -> MATLAB Function/1(x)
  VVC_1547_CATB/1(a) -> MATLAB Function/2(a)
  VVC_1547_CATB/2(b) -> MATLAB Function/3(b)
  VVC_1547_CATA/1(c) -> MATLAB Function/4(c)
  VVC_1547_CATA/2(d) -> MATLAB Function/5(d)
  VVC_EPRI_CS1/1(e) -> MATLAB Function/6(e)
  VVC_EPRI_CS1/2(f) -> MATLAB Function/7(f)
  VVC_EPRI_CS2/1(g) -> MATLAB Function/8(g)
  VVC_EPRI_CS2/2(h) -> MATLAB Function/9(h)
  VVC_CS3/1(Out1) -> MATLAB Function/10(i)
  VVC_CS3/2(Out2) -> MATLAB Function/11(j)
  VVC_CS2/1(k) -> MATLAB Function/12(k)
  VVC_CS2/2(l) -> MATLAB Function/13(l)
  VVC_CS4/1(m) -> MATLAB Function/14(m)
  VVC_CS4/2(n) -> MATLAB Function/15(n)
  VVC_CCC/1(o) -> MATLAB Function/16(o)
  VVC_CCC/2(p) -> MATLAB Function/17(p)
  VVC_CCC44/2(p) -> Bus Creator/2
  VVC_CCC44/1(o) -> Bus Creator/1
  VVC_CCCOpt/1(o) -> Bus Creator1/1
  VVC_CCCOpt/2(p) -> Bus Creator1/2
  Constant/1 -> Subtract/2
  Switch5/1 -> Memory1/1
  Set-Reset Flip-Flop1/2 -> Discrete-Time Integrator/2
  Constant2/1 -> Switch4/3
  Constant1/1 -> Product1/3
  Switch/1 -> Bus Selector/1
  Product1/1 -> Tanh/1
  Constant3/1 -> Discrete-Time Integrator/1
  Subtract/1 -> Abs/1
  Bus Creator/1 -> Switch/3
  Product/1 -> Switch5/3
  Switch4/1 -> Set-Reset Flip-Flop1/1
  Bus Selector/2 -> VV/3  "<signal2>"
  Set-Reset Flip-Flop1/1 -> [SRS], Scope/1
  Step1/1 -> Switch4/2
  Memory1/1 -> Switch5/1
  Gain9/1 -> Product/2, Switch3/3  "Iqvv"
  Derivative/1 -> Scope1/1, Compare To Constant1/1
  In1/1 -> VV/1, [Vb], Compare To Constant/1, Derivative/1
  Tanh/1 -> Switch5/2, Product/1
  Bus Creator1/1 -> Switch/1
  Abs/1 -> Product1/2
  Compare To Constant1/1 -> Set-Reset Flip-Flop1/2
  Saturation1/1 -> Gain9/1
  [Vb] -> Subtract/1
  Compare To Constant/1 -> Switch4/1
  [SRS] -> Switch/2
  Discrete-Time Integrator/1 -> Product1/1
  VV/1 -> Saturation1/1
  Bus Selector/1 -> VV/2  "<signal1>"
  Memory3/1 -> Switch3/1
  [SRS] -> Switch3/2
  Switch3/1 -> Iqvv/1, Memory3/1  "Iqvv"

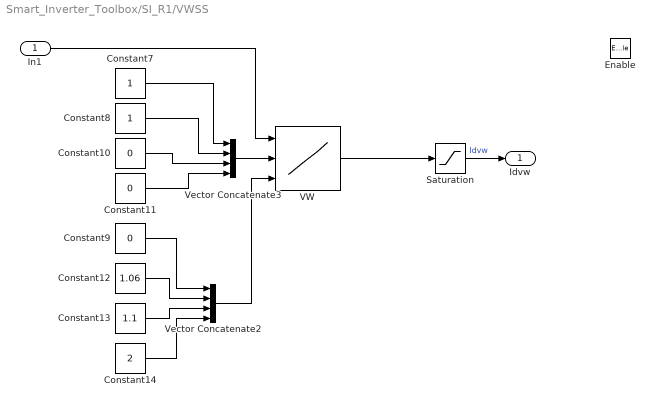
== system Smart_Inverter_Toolbox/SI_R1/VWSS ==
  In1 : Inport
  Enable : EnablePort
  Constant10 : Constant  Value=0
  Constant11 : Constant  Value=0
  Constant12 : Constant  Value=1.06
  Constant13 : Constant  Value=1.1
  Constant14 : Constant  Value=2
  Constant7 : Constant
  Constant8 : Constant
  Constant9 : Constant  Value=0
  Saturation : Saturate  UpperLimit=1  LowerLimit=0
  VW : Lookup_n-D  NumberOfTableDimensions=1  BreakpointsForDimension1Source=Input port  BreakpointsForDimension1=[-5:5]  TableSource=Input port  Table=tanh([-5:5])  ExtrapMethod=Clip  InternalRulePriority=Speed  RndMeth=Simplest
      settings: InputPortMap=u0,p221,p5
  Vector Concatenate2 : Concatenate  NumInputs=4
  Vector Concatenate3 : Concatenate  NumInputs=4
  Idvw : Outport
  wires:
  Constant7/1 -> Vector Concatenate3/1
  Constant14/1 -> Vector Concatenate2/4
  Constant11/1 -> Vector Concatenate3/4
  Constant10/1 -> Vector Concatenate3/3
  Constant8/1 -> Vector Concatenate3/2
  Constant13/1 -> Vector Concatenate2/3
  Constant12/1 -> Vector Concatenate2/2
  Vector Concatenate3/1 -> VW/2
  Constant9/1 -> Vector Concatenate2/1
  In1/1 -> VW/1
  Saturation/1 -> Idvw/1  "Idvw"
  Vector Concatenate2/1 -> VW/3
  VW/1 -> Saturation/1

== system Smart_Inverter_Toolbox/SI_R1/VVSS/VVC_1547_CATA ==
  Constant1 : Constant  Value=0.22
  Constant10 : Constant  Value=0.1
  Constant11 : Constant  Value=0.9
  Constant14 : Constant  Value=1.1
  Constant2 : Constant  Value=-0.22
  Constant24 : Constant  Value=2
  Constant3 : Constant  Value=-0.22
  Constant4 : Constant  Value=2.1
  Constant5 : Constant  Value=0
  Constant9 : Constant  Value=0.22
  Vector Concatenate1 : Concatenate  NumInputs=6
  Vector Concatenate2 : Concatenate  NumInputs=6
  c : Outport
  d : Outport  Port=2
  wires:
  Constant2/1 -> Vector Concatenate1/4
  Constant11/1 -> Vector Concatenate2/3
  Constant10/1 -> Vector Concatenate2/2
  Constant5/1 -> Vector Concatenate2/1
  Constant4/1 -> Vector Concatenate2/6
  Constant3/1 -> Vector Concatenate1/6, Vector Concatenate1/5
  Constant1/1 -> Vector Concatenate1/3
  Constant14/1 -> Vector Concatenate2/4
  Vector Concatenate1/1 -> c/1  "T"
  Constant9/1 -> Vector Concatenate1/1, Vector Concatenate1/2
  Vector Concatenate2/1 -> d/1  "BP"
  Constant24/1 -> Vector Concatenate2/5

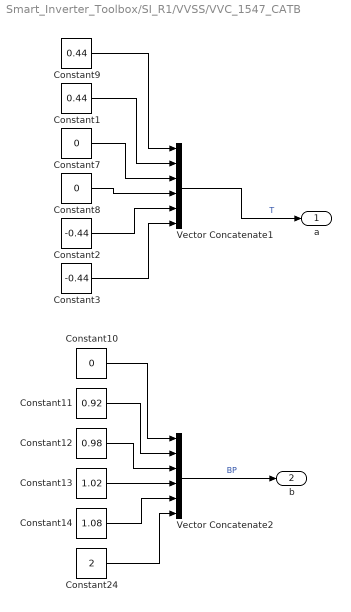
== system Smart_Inverter_Toolbox/SI_R1/VVSS/VVC_1547_CATB ==
  Constant1 : Constant  Value=0.44
  Constant10 : Constant  Value=0
  Constant11 : Constant  Value=0.92
  Constant12 : Constant  Value=0.98
  Constant13 : Constant  Value=1.02
  Constant14 : Constant  Value=1.08
  Constant2 : Constant  Value=-0.44
  Constant24 : Constant  Value=2
  Constant3 : Constant  Value=-0.44
  Constant7 : Constant  Value=0
  Constant8 : Constant  Value=0
  Constant9 : Constant  Value=0.44
  Vector Concatenate1 : Concatenate  NumInputs=6
  Vector Concatenate2 : Concatenate  NumInputs=6
  a : Outport
  b : Outport  Port=2
  wires:
  Vector Concatenate1/1 -> a/1  "T"
  Vector Concatenate2/1 -> b/1  "BP"
  Constant9/1 -> Vector Concatenate1/1
  Constant7/1 -> Vector Concatenate1/3
  Constant3/1 -> Vector Concatenate1/6
  Constant1/1 -> Vector Concatenate1/2
  Constant11/1 -> Vector Concatenate2/2
  Constant10/1 -> Vector Concatenate2/1
  Constant12/1 -> Vector Concatenate2/3
  Constant24/1 -> Vector Concatenate2/6
  Constant2/1 -> Vector Concatenate1/5
  Constant14/1 -> Vector Concatenate2/5
  Constant8/1 -> Vector Concatenate1/4
  Constant13/1 -> Vector Concatenate2/4

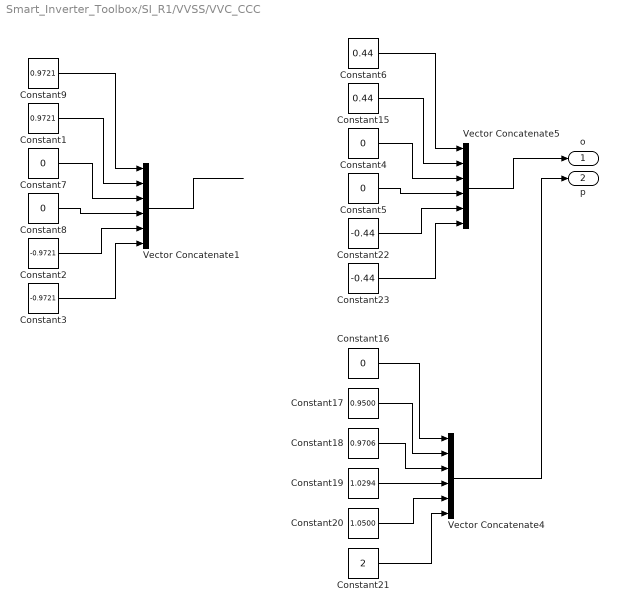
== system Smart_Inverter_Toolbox/SI_R1/VVSS/VVC_CCC ==
  Constant1 : Constant  Value=0.9721
  Constant15 : Constant  Value=0.44
  Constant{4..5,7..8,16} (5 alike) : Constant  Value=0
  Constant17 : Constant  Value=0.9500
  Constant18 : Constant  Value=0.9706
  Constant19 : Constant  Value=1.0294
  Constant2 : Constant  Value=-0.9721
  Constant20 : Constant  Value=1.0500
  Constant21 : Constant  Value=2
  Constant22 : Constant  Value=-0.44
  Constant23 : Constant  Value=-0.44
  Constant3 : Constant  Value=-0.9721
  Constant6 : Constant  Value=0.44
  Constant9 : Constant  Value=0.9721
  Vector Concatenate1 : Concatenate  NumInputs=6
  Vector Concatenate4 : Concatenate  NumInputs=6
  Vector Concatenate5 : Concatenate  NumInputs=6
  o : Outport
  p : Outport  Port=2
  wires:
  Vector Concatenate5/1 -> o/1
  Vector Concatenate4/1 -> p/1
  Constant4/1 -> Vector Concatenate5/3
  Constant16/1 -> Vector Concatenate4/1
  Constant21/1 -> Vector Concatenate4/6
  Constant23/1 -> Vector Concatenate5/6
  Constant5/1 -> Vector Concatenate5/4
  Constant17/1 -> Vector Concatenate4/2
  Constant6/1 -> Vector Concatenate5/1
  Constant18/1 -> Vector Concatenate4/3
  Constant22/1 -> Vector Concatenate5/5
  Constant20/1 -> Vector Concatenate4/5
  Constant19/1 -> Vector Concatenate4/4
  Constant15/1 -> Vector Concatenate5/2
  Constant1/1 -> Vector Concatenate1/2
  Constant2/1 -> Vector Concatenate1/5
  Constant9/1 -> Vector Concatenate1/1
  Constant8/1 -> Vector Concatenate1/4
  Constant3/1 -> Vector Concatenate1/6
  Constant7/1 -> Vector Concatenate1/3
  Vector Concatenate1/1 -> ?

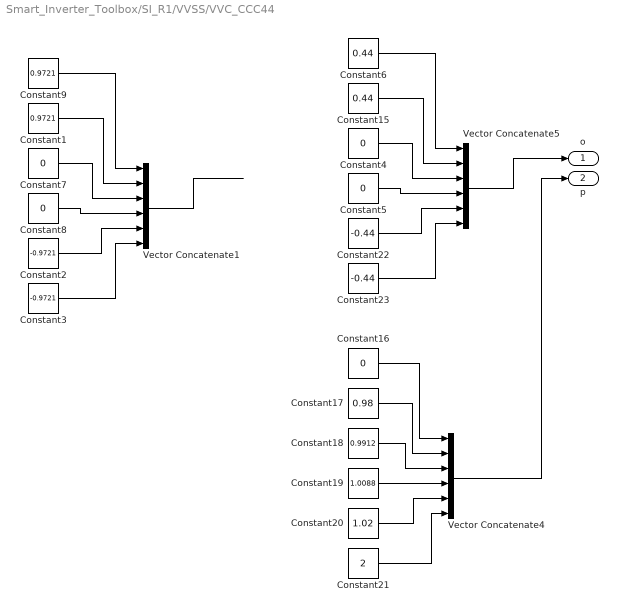
== system Smart_Inverter_Toolbox/SI_R1/VVSS/VVC_CCC44 ==
  Constant1 : Constant  Value=0.9721
  Constant15 : Constant  Value=0.44
  Constant{4..5,7..8,16} (5 alike) : Constant  Value=0
  Constant17 : Constant  Value=0.98
  Constant18 : Constant  Value=0.9912
  Constant19 : Constant  Value=1.0088
  Constant2 : Constant  Value=-0.9721
  Constant20 : Constant  Value=1.02
  Constant21 : Constant  Value=2
  Constant22 : Constant  Value=-0.44
  Constant23 : Constant  Value=-0.44
  Constant3 : Constant  Value=-0.9721
  Constant6 : Constant  Value=0.44
  Constant9 : Constant  Value=0.9721
  Vector Concatenate1 : Concatenate  NumInputs=6
  Vector Concatenate4 : Concatenate  NumInputs=6
  Vector Concatenate5 : Concatenate  NumInputs=6
  o : Outport
  p : Outport  Port=2
  wires:
  Vector Concatenate1/1 -> ?
  Constant7/1 -> Vector Concatenate1/3
  Constant3/1 -> Vector Concatenate1/6
  Constant8/1 -> Vector Concatenate1/4
  Constant9/1 -> Vector Concatenate1/1
  Constant2/1 -> Vector Concatenate1/5
  Constant1/1 -> Vector Concatenate1/2
  Constant15/1 -> Vector Concatenate5/2
  Constant19/1 -> Vector Concatenate4/4
  Constant20/1 -> Vector Concatenate4/5
  Constant22/1 -> Vector Concatenate5/5
  Constant18/1 -> Vector Concatenate4/3
  Constant6/1 -> Vector Concatenate5/1
  Constant17/1 -> Vector Concatenate4/2
  Constant5/1 -> Vector Concatenate5/4
  Constant23/1 -> Vector Concatenate5/6
  Constant21/1 -> Vector Concatenate4/6
  Constant16/1 -> Vector Concatenate4/1
  Constant4/1 -> Vector Concatenate5/3
  Vector Concatenate4/1 -> p/1
  Vector Concatenate5/1 -> o/1

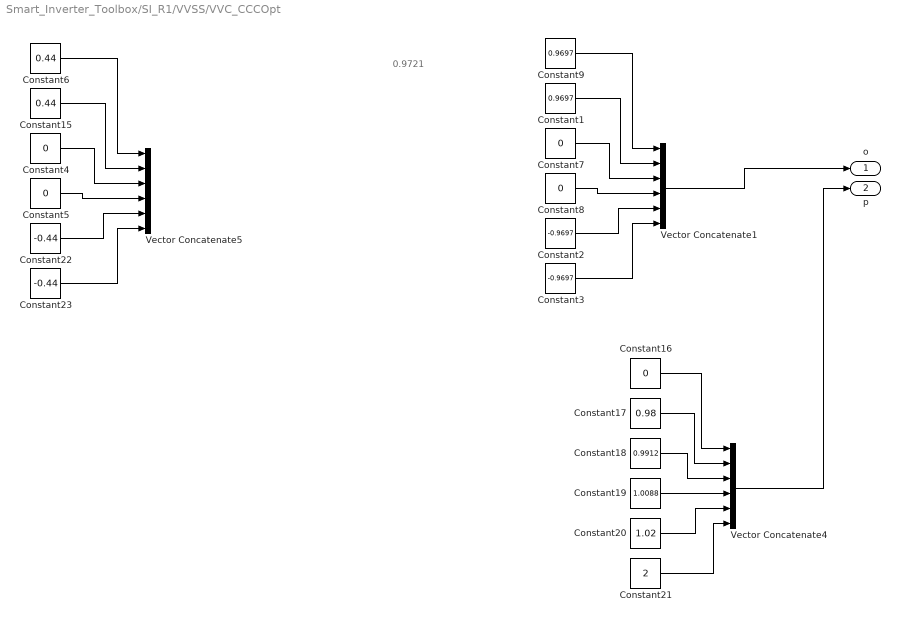
== system Smart_Inverter_Toolbox/SI_R1/VVSS/VVC_CCCOpt ==
  note: 0.9721
  Constant1 : Constant  Value=0.9697
  Constant15 : Constant  Value=0.44
  Constant{4..5,7..8,16} (5 alike) : Constant  Value=0
  Constant17 : Constant  Value=0.98
  Constant18 : Constant  Value=0.9912
  Constant19 : Constant  Value=1.0088
  Constant2 : Constant  Value=-0.9697
  Constant20 : Constant  Value=1.02
  Constant21 : Constant  Value=2
  Constant22 : Constant  Value=-0.44
  Constant23 : Constant  Value=-0.44
  Constant3 : Constant  Value=-0.9697
  Constant6 : Constant  Value=0.44
  Constant9 : Constant  Value=0.9697
  Vector Concatenate1 : Concatenate  NumInputs=6
  Vector Concatenate4 : Concatenate  NumInputs=6
  Vector Concatenate5 : Concatenate  NumInputs=6
  o : Outport
  p : Outport  Port=2
  wires:
  Vector Concatenate1/1 -> o/1
  Vector Concatenate4/1 -> p/1
  Constant4/1 -> Vector Concatenate5/3
  Constant16/1 -> Vector Concatenate4/1
  Constant21/1 -> Vector Concatenate4/6
  Constant23/1 -> Vector Concatenate5/6
  Constant5/1 -> Vector Concatenate5/4
  Constant17/1 -> Vector Concatenate4/2
  Constant6/1 -> Vector Concatenate5/1
  Constant18/1 -> Vector Concatenate4/3
  Constant22/1 -> Vector Concatenate5/5
  Constant20/1 -> Vector Concatenate4/5
  Constant19/1 -> Vector Concatenate4/4
  Constant15/1 -> Vector Concatenate5/2
  Constant1/1 -> Vector Concatenate1/2
  Constant2/1 -> Vector Concatenate1/5
  Constant9/1 -> Vector Concatenate1/1
  Constant8/1 -> Vector Concatenate1/4
  Constant3/1 -> Vector Concatenate1/6
  Constant7/1 -> Vector Concatenate1/3

== system Smart_Inverter_Toolbox/SI_R1/VVSS/VVC_CS2 ==
  Constant12 : Constant  Value=2
  Constant13 : Constant  Value=-1
  Constant15 : Constant  Value=2.1
  Constant16 : Constant  Value=0
  Constant17 : Constant
  Constant4 : Constant
  Constant5 : Constant  Value=0.1
  Constant6 : Constant  Value=0.95
  Constant7 : Constant  Value=1.05
  Constant8 : Constant  Value=-1
  Vector Concatenate3 : Concatenate  NumInputs=6
  Vector Concatenate4 : Concatenate  NumInputs=6
  k : Outport
  l : Outport  Port=2
  wires:
  Constant6/1 -> Vector Concatenate4/3
  Constant7/1 -> Vector Concatenate4/4
  Constant15/1 -> Vector Concatenate4/6
  Constant5/1 -> Vector Concatenate4/2
  Constant12/1 -> Vector Concatenate4/5
  Constant13/1 -> Vector Concatenate3/5, Vector Concatenate3/6
  Vector Concatenate3/1 -> k/1  "T"
  Constant17/1 -> Vector Concatenate3/1, Vector Concatenate3/2
  Constant16/1 -> Vector Concatenate4/1
  Constant4/1 -> Vector Concatenate3/3
  Constant8/1 -> Vector Concatenate3/4
  Vector Concatenate4/1 -> l/1  "BP"

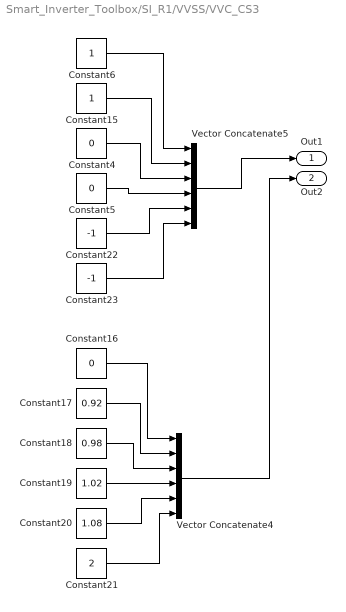
== system Smart_Inverter_Toolbox/SI_R1/VVSS/VVC_CS3 ==
  Constant15 : Constant
  Constant16 : Constant  Value=0
  Constant17 : Constant  Value=0.92
  Constant18 : Constant  Value=0.98
  Constant19 : Constant  Value=1.02
  Constant20 : Constant  Value=1.08
  Constant21 : Constant  Value=2
  Constant22 : Constant  Value=-1
  Constant23 : Constant  Value=-1
  Constant4 : Constant  Value=0
  Constant5 : Constant  Value=0
  Constant6 : Constant
  Vector Concatenate4 : Concatenate  NumInputs=6
  Vector Concatenate5 : Concatenate  NumInputs=6
  Out1 : Outport
  Out2 : Outport  Port=2
  wires:
  Constant15/1 -> Vector Concatenate5/2
  Constant19/1 -> Vector Concatenate4/4
  Constant20/1 -> Vector Concatenate4/5
  Constant22/1 -> Vector Concatenate5/5
  Constant18/1 -> Vector Concatenate4/3
  Constant6/1 -> Vector Concatenate5/1
  Constant17/1 -> Vector Concatenate4/2
  Constant5/1 -> Vector Concatenate5/4
  Constant23/1 -> Vector Concatenate5/6
  Constant21/1 -> Vector Concatenate4/6
  Constant16/1 -> Vector Concatenate4/1
  Constant4/1 -> Vector Concatenate5/3
  Vector Concatenate4/1 -> Out2/1
  Vector Concatenate5/1 -> Out1/1

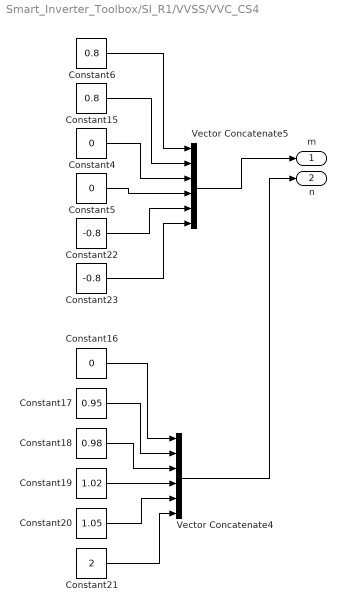
== system Smart_Inverter_Toolbox/SI_R1/VVSS/VVC_CS4 ==
  Constant15 : Constant  Value=0.8
  Constant16 : Constant  Value=0
  Constant17 : Constant  Value=0.95
  Constant18 : Constant  Value=0.98
  Constant19 : Constant  Value=1.02
  Constant20 : Constant  Value=1.05
  Constant21 : Constant  Value=2
  Constant22 : Constant  Value=-0.8
  Constant23 : Constant  Value=-0.8
  Constant4 : Constant  Value=0
  Constant5 : Constant  Value=0
  Constant6 : Constant  Value=0.8
  Vector Concatenate4 : Concatenate  NumInputs=6
  Vector Concatenate5 : Concatenate  NumInputs=6
  m : Outport
  n : Outport  Port=2
  wires:
  Constant15/1 -> Vector Concatenate5/2
  Constant19/1 -> Vector Concatenate4/4
  Constant20/1 -> Vector Concatenate4/5
  Constant22/1 -> Vector Concatenate5/5
  Constant18/1 -> Vector Concatenate4/3
  Constant6/1 -> Vector Concatenate5/1
  Constant17/1 -> Vector Concatenate4/2
  Constant5/1 -> Vector Concatenate5/4
  Constant23/1 -> Vector Concatenate5/6
  Constant21/1 -> Vector Concatenate4/6
  Constant16/1 -> Vector Concatenate4/1
  Constant4/1 -> Vector Concatenate5/3
  Vector Concatenate4/1 -> n/1
  Vector Concatenate5/1 -> m/1

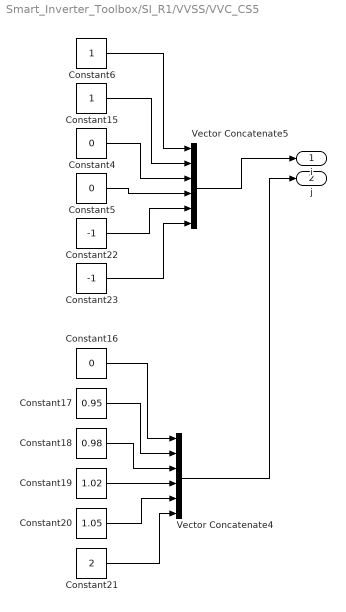
== system Smart_Inverter_Toolbox/SI_R1/VVSS/VVC_CS5 ==
  Constant15 : Constant
  Constant16 : Constant  Value=0
  Constant17 : Constant  Value=0.95
  Constant18 : Constant  Value=0.98
  Constant19 : Constant  Value=1.02
  Constant20 : Constant  Value=1.05
  Constant21 : Constant  Value=2
  Constant22 : Constant  Value=-1
  Constant23 : Constant  Value=-1
  Constant4 : Constant  Value=0
  Constant5 : Constant  Value=0
  Constant6 : Constant
  Vector Concatenate4 : Concatenate  NumInputs=6
  Vector Concatenate5 : Concatenate  NumInputs=6
  i : Outport
  j : Outport  Port=2
  wires:
  Constant15/1 -> Vector Concatenate5/2
  Constant19/1 -> Vector Concatenate4/4
  Constant20/1 -> Vector Concatenate4/5
  Constant22/1 -> Vector Concatenate5/5
  Constant18/1 -> Vector Concatenate4/3
  Constant6/1 -> Vector Concatenate5/1
  Constant17/1 -> Vector Concatenate4/2
  Constant5/1 -> Vector Concatenate5/4
  Constant23/1 -> Vector Concatenate5/6
  Constant21/1 -> Vector Concatenate4/6
  Constant16/1 -> Vector Concatenate4/1
  Constant4/1 -> Vector Concatenate5/3
  Vector Concatenate4/1 -> j/1
  Vector Concatenate5/1 -> i/1

== system Smart_Inverter_Toolbox/SI_R1/VVSS/VVC_EPRI_CS1 ==
  Constant1 : Constant  Value=0.44
  Constant10 : Constant  Value=0.1
  Constant11 : Constant  Value=0.9
  Constant14 : Constant  Value=1.1
  Constant2 : Constant  Value=-0.44
  Constant24 : Constant  Value=2
  Constant3 : Constant  Value=-0.44
  Constant4 : Constant  Value=2.1
  Constant5 : Constant  Value=0
  Constant9 : Constant  Value=0.44
  Vector Concatenate1 : Concatenate  NumInputs=6
  Vector Concatenate2 : Concatenate  NumInputs=6
  e : Outport
  f : Outport  Port=2
  wires:
  Constant24/1 -> Vector Concatenate2/5
  Constant2/1 -> Vector Concatenate1/4
  Constant14/1 -> Vector Concatenate2/4
  Constant10/1 -> Vector Concatenate2/2
  Constant11/1 -> Vector Concatenate2/3
  Constant1/1 -> Vector Concatenate1/3
  Constant3/1 -> Vector Concatenate1/5, Vector Concatenate1/6
  Constant9/1 -> Vector Concatenate1/1, Vector Concatenate1/2
  Vector Concatenate2/1 -> f/1  "BP"
  Vector Concatenate1/1 -> e/1  "T"
  Constant4/1 -> Vector Concatenate2/6
  Constant5/1 -> Vector Concatenate2/1

== system Smart_Inverter_Toolbox/SI_R1/VVSS/VVC_EPRI_CS2 ==
  Constant12 : Constant  Value=2
  Constant13 : Constant  Value=-0.44
  Constant15 : Constant  Value=2.1
  Constant16 : Constant  Value=0
  Constant17 : Constant  Value=0.44
  Constant4 : Constant  Value=0.44
  Constant5 : Constant  Value=0.1
  Constant6 : Constant  Value=0.95
  Constant7 : Constant  Value=1.05
  Constant8 : Constant  Value=-0.44
  Vector Concatenate3 : Concatenate  NumInputs=6
  Vector Concatenate4 : Concatenate  NumInputs=6
  g : Outport
  h : Outport  Port=2
  wires:
  Constant6/1 -> Vector Concatenate4/3
  Constant7/1 -> Vector Concatenate4/4
  Constant15/1 -> Vector Concatenate4/6
  Constant5/1 -> Vector Concatenate4/2
  Constant12/1 -> Vector Concatenate4/5
  Constant13/1 -> Vector Concatenate3/5, Vector Concatenate3/6
  Vector Concatenate3/1 -> g/1  "T"
  Constant17/1 -> Vector Concatenate3/1, Vector Concatenate3/2
  Constant16/1 -> Vector Concatenate4/1
  Constant4/1 -> Vector Concatenate3/3
  Constant8/1 -> Vector Concatenate3/4
  Vector Concatenate4/1 -> h/1  "BP"

== matlab function Smart_Inverter_Toolbox/SI_R1/MATLAB Function ==
  data: rpm input; ECPF output; pps input; vwm input; EVV output; ECRP output; EPVS output; pvmps output; spmps output; EAPP output; ERPP output; ppmps output; cpfmps output
function [ECPF,EVV,ECRP,EPVS,pvmps,spmps,EAPP,ERPP,ppmps,cpfmps] = ModeLogic(rpm,pps,vwm)

ECPF = 0;
EVV  = 0;
ECRP = 0;
EPVS = 0;
pvmps = 0;
spmps = 0;
EAPP = 0;
ERPP = 0;
ppmps = 0;
cpfmps = 0;

switch rpm
    
    case 1
        ECPF=1;
        EPVS=1;
        pvmps=1;
        spmps=1;   
        cpfmps=1;

        if vwm==1
            cpfmps=2;
        end

    case 2
        EVV=1;

        switch pps
            case 1
                EAPP=1;
                ppmps=1;
                spmps=2;

                if vwm==1
                    ppmps=3;        
                end

            case 2
                ERPP=1;
                ppmps=1;
                spmps=3;

                if vwm==1
                    ppmps=3;        
                end

            case 3
                EPVS=1;
                pvmps=2;
                spmps=1;

                if vwm==1
                    pvmps=3;
                end                
        end

    case 3
        ECRP=1;
        ERPP=1;
        ppmps=2;
        spmps=3;

        if vwm==1
            ppmps=4;
        end

    otherwise
      
end

if vwm==2
    spmps=4;
end

end

== matlab function Smart_Inverter_Toolbox/SI_R1/VVSS/MATLAB Function ==
  data: x input; a input; T output; b input; bp output; c input; d input; e input; f input; g input; h input; i input; j input; k input; l input; m input; n input; o input; p input
function [T, bp] = fcn(x, a, b, c, d, e, f, g, h, i, j, k, l, m, n, o, p)


switch x
    
    case 1
        T=a;
        bp=b;
    case 2
        T=c;
        bp=d;
    case 3
        T=e;
        bp=f;
    case 4
        T=g;
        bp=h;
    case 5
        T=i;
        bp=j;
    case 6
        T=k;
        bp=l;
    case 7
        T=m;
        bp=n;
    case 8
        T=o;
        bp=p;

    otherwise
        T=a;
        bp=b;
        
end
